simulink subsystem "Mk2Transmission"  (R2024a)
settings: Solver=VariableStepAuto  StartTime=0.0  StopTime=10.0  RelTol=1e-3
undefined symbols (not defined in the file): Motor1, Motor2, Motor3, Transmission1_Stage1, Transmission1_Stage2, Transmission2_Stage1, Transmission2_Stage2, Transmission3_Stage1
libraries: sdl_lib x4, fl_lib x3
settings Model: DataDictionary=neck_mk3.sldd  EnableAccessToBaseWorkspace=off  Creator=upattacini  LastModifiedBy=upattacini
settings RTWCC: GPUComputeCapability=3.5

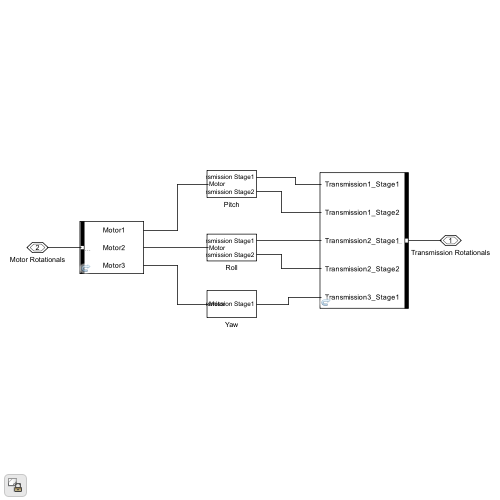
[thumbnail: Simulink's stored preview of the top-level diagram]
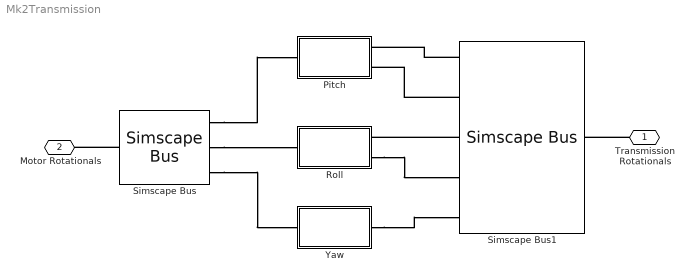
== system Mk2Transmission ==
  Pitch : Subsystem
  Roll : Subsystem
  Simscape Bus : SimscapeBus  HierarchyStrings=Motor1;Motor2;Motor3  ConnectionType=Bus: Physical_MotorRotationals
  Simscape Bus1 : SimscapeBus  HierarchyStrings=Transmission1_Stage1;Transmission1_Stage2;Transmission2_Stage1;Transmission2_Stage2;Transmission3_Stage1  ConnectionType=Bus: Physical_TransmissionRotationals
  Yaw : Subsystem
  Transmission Rotationals : PMIOPort  Side=Right  ConnectionType=Bus: Physical_TransmissionRotationals
  Motor Rotationals : PMIOPort  Port=2  Side=Left  ConnectionType=Bus: Physical_MotorRotationals
  connections:
  Simscape Bus/RConn1 -- Motor Rotationals/RConn1
  Simscape Bus/LConn3 -- Yaw/LConn1
  Simscape Bus/LConn1 -- Pitch/LConn1
  Simscape Bus/LConn2 -- Roll/LConn1
  Simscape Bus1/LConn1 -- Pitch/RConn1
  Simscape Bus1/LConn2 -- Pitch/RConn2
  Simscape Bus1/LConn3 -- Roll/RConn1
  Roll/RConn2 -- Simscape Bus1/LConn4
  Yaw/RConn1 -- Simscape Bus1/LConn5
  Transmission Rotationals/RConn1 -- Simscape Bus1/RConn1

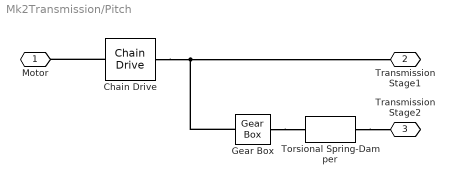
== system Mk2Transmission/Pitch ==
  Chain Drive : sdl_lib/Couplings & Drives/Chain Drive  chain_model=sdl.enum.chain_model.flexible  radius_a=5.82 mm  radius_b=9.055 mm  slack=0 mm  k_chain=243.923187368682*100 N/m  mu_visc_chain=24.3923187368682*100 N*s/m  mu_visc_a=0 N*m*s/rad  mu_visc_b=0 N*m*s/rad  breakable=sdl.enum.max_tension.off  F_max=1e6 N  x_specify=off  x_priority=High  x=0 mm  x_nominal_specify=off  x_nominal_value=1  x_nominal_unit=mm
      settings: InternalSimscapePortConfiguration="{\"Bottom\":[],\"Left\":[{\"id\":\"A\",\"label\":\"A\",\"type\":\"foundation.mechanical.rotational.rotational\"}],\"Right\":[{\"id\":\"B\",\"label\":\"B\",\"type\":\"foundation.mechanical.rotational.rotational\"}],\"Top\":[]}"
  Gear Box : fl_lib/Mechanical/Mechanisms/Gear Box  ratio=100  t_in_specify=off  t_in_priority=None  t_in=0 N*m  t_in_nominal_specify=off  t_in_nominal_value=1  t_in_nominal_unit=N*m  t_out_specify=off  t_out_priority=None  t_out=0 N*m  t_out_nominal_specify=off  t_out_nominal_value=1  t_out_nominal_unit=N*m
  Torsional Spring-Damper : sdl_lib/Couplings & Drives/Torsional Spring-Damper  k=200*100 N*m/rad  mu_visc=20*100 N*m*s/rad  trq_coulomb=0 N*m  static_kinetic_ratio=1.1  w_tol=0.001 rad/s  model_hardstop=sdl.enum.hardStopOffOn.off  upper_bound=10 deg  lower_bound=-10 deg  hardstop_model=simscape.enum.hardstop.smooth  k_endstop=1e6 N*m/rad  D_endstop=10 N*m*s/rad  transition=0.001 rad  coeff_rest=0.7  w_tol_hardstop=0.1 rad/s  trq_tol=0.001 N*m  x0=0 deg
      settings: InternalSimscapePortConfiguration="{\"Bottom\":[],\"Left\":[{\"id\":\"R\",\"label\":\"R\",\"type\":\"foundation.mechanical.rotational.rotational\"}],\"Right\":[{\"id\":\"C\",\"label\":\"C\",\"type\":\"foundation.mechanical.rotational.rotational\"}],\"Top\":[]}"
  Motor : PMIOPort  Side=Left
  Transmission Stage1 : PMIOPort  Port=2  Side=Right
  Transmission Stage2 : PMIOPort  Port=3  Side=Right
  connections:
  Gear Box/RConn1 -- Torsional Spring-Damper/LConn1
  Chain Drive/RConn1 -- Gear Box/LConn1 -- Transmission Stage1/RConn1
  Chain Drive/LConn1 -- Motor/RConn1
  Torsional Spring-Damper/RConn1 -- Transmission Stage2/RConn1

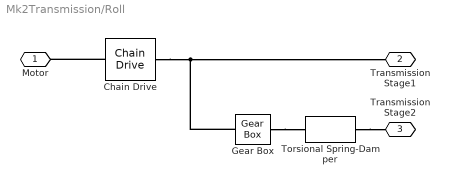
== system Mk2Transmission/Roll ==
  Chain Drive : sdl_lib/Couplings & Drives/Chain Drive  chain_model=sdl.enum.chain_model.flexible  radius_a=5.82 mm  radius_b=9.055 mm  slack=0 mm  k_chain=243.923187368682*100 N/m  mu_visc_chain=24.3923187368682*100 N*s/m  mu_visc_a=0 N*m*s/rad  mu_visc_b=0 N*m*s/rad  breakable=sdl.enum.max_tension.off  F_max=1e6 N  x_specify=off  x_priority=High  x=0 mm  x_nominal_specify=off  x_nominal_value=1  x_nominal_unit=mm
      settings: InternalSimscapePortConfiguration="{\"Bottom\":[],\"Left\":[{\"id\":\"A\",\"label\":\"A\",\"type\":\"foundation.mechanical.rotational.rotational\"}],\"Right\":[{\"id\":\"B\",\"label\":\"B\",\"type\":\"foundation.mechanical.rotational.rotational\"}],\"Top\":[]}"
  Gear Box : fl_lib/Mechanical/Mechanisms/Gear Box  ratio=100  t_in_specify=off  t_in_priority=None  t_in=0 N*m  t_in_nominal_specify=off  t_in_nominal_value=1  t_in_nominal_unit=N*m  t_out_specify=off  t_out_priority=None  t_out=0 N*m  t_out_nominal_specify=off  t_out_nominal_value=1  t_out_nominal_unit=N*m
  Torsional Spring-Damper : sdl_lib/Couplings & Drives/Torsional Spring-Damper  k=200*100 N*m/rad  mu_visc=20*100 N*m*s/rad  trq_coulomb=0 N*m  static_kinetic_ratio=1.1  w_tol=0.001 rad/s  model_hardstop=sdl.enum.hardStopOffOn.off  upper_bound=10 deg  lower_bound=-10 deg  hardstop_model=simscape.enum.hardstop.smooth  k_endstop=1e6 N*m/rad  D_endstop=10 N*m*s/rad  transition=0.001 rad  coeff_rest=0.7  w_tol_hardstop=0.1 rad/s  trq_tol=0.001 N*m  x0=0 deg
      settings: InternalSimscapePortConfiguration="{\"Bottom\":[],\"Left\":[{\"id\":\"R\",\"label\":\"R\",\"type\":\"foundation.mechanical.rotational.rotational\"}],\"Right\":[{\"id\":\"C\",\"label\":\"C\",\"type\":\"foundation.mechanical.rotational.rotational\"}],\"Top\":[]}"
  Motor : PMIOPort  Side=Left
  Transmission Stage1 : PMIOPort  Port=2  Side=Right
  Transmission Stage2 : PMIOPort  Port=3  Side=Right
  connections:
  Torsional Spring-Damper/RConn1 -- Transmission Stage2/RConn1
  Gear Box/RConn1 -- Torsional Spring-Damper/LConn1
  Chain Drive/LConn1 -- Motor/RConn1
  Chain Drive/RConn1 -- Transmission Stage1/RConn1 -- Gear Box/LConn1

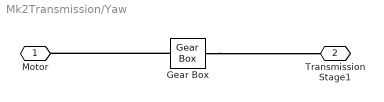
== system Mk2Transmission/Yaw ==
  Gear Box : fl_lib/Mechanical/Mechanisms/Gear Box  ratio=100  t_in_specify=off  t_in_priority=None  t_in=0 N*m  t_in_nominal_specify=off  t_in_nominal_value=1  t_in_nominal_unit=N*m  t_out_specify=off  t_out_priority=None  t_out=0 N*m  t_out_nominal_specify=off  t_out_nominal_value=1  t_out_nominal_unit=N*m
  Motor : PMIOPort  Side=Left
  Transmission Stage1 : PMIOPort  Port=2  Side=Right
  connections:
  Gear Box/LConn1 -- Motor/RConn1
  Gear Box/RConn1 -- Transmission Stage1/RConn1
